simulink model "Vicon_Visualization"  (Simulink 9.1)
settings: Solver=FixedStepDiscrete  StartTime=0.0  StopTime=inf  FixedStep=0.001  RelTol=1e-3  EnableMultiTasking=on
undefined symbols (not defined in the file): localhost
libraries: quarc_library x6
settings Model: Creator=glai  LastModifiedBy=user  SimulationMode=external  ExtModeTrigDuration=5000
settings SolverCC: PositivePriorityOrder=on
settings DataIOCC: LimitDataPoints=on
settings OptimizationCC: LifeSpan=auto
settings DebuggingCC: UnderspecifiedInitializationDetection=Simplified  MergeDetectMultiDrivingBlocksExec=error  SolverPrmCheckMsg=warning
settings HardwareCC: ProdBitPerPointer=64  ProdBitPerSizeT=64  ProdBitPerPtrDiffT=64  ProdLargestAtomicFloat=Float  ProdIntDivRoundTo=Zero  ProdEndianess=LittleEndian  ProdWordSize=64  ProdHWDeviceType=Intel->x86-64 (Windows64)
settings RTWCC: Description=QUARC Win64 Target Using Toolchain  SystemTargetFile=quarc_win64.tlc  TemplateMakefile=quarc_default_tmf  Toolchain=QUARC win64 | nmake (64-bit Windows)  BuildConfiguration=Faster Runs
settings STFCustomTargetCC: ConcurrentExecutionCompliant=on  UseToolchainInfoCompliant=on  SystemTargetFile=quarc_win64.tlc
settings GRTTargetCC: ParMdlRefBuildCompliant=off  CompOptLevelCompliant=off  MatFileLogging=off  CPPClassGenCompliant=off  ExtMode=on  ExtModeMexFile=quarc_comm  ExtModeMexArgs='-w -d %d -uri %u', 'shmem://%m:1?timeout=10'
settings ConfigComp: CovSFcnEnable=off

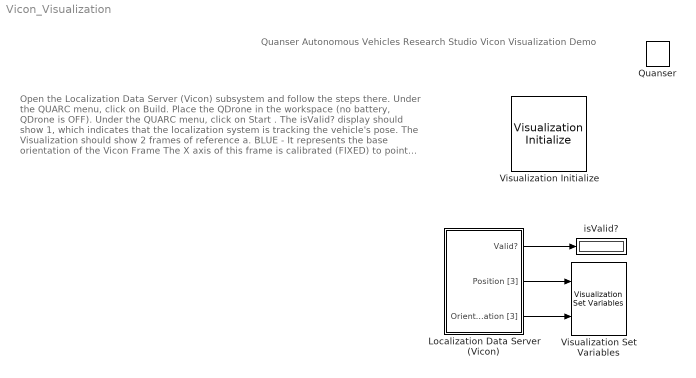
== system Vicon_Visualization ==
  note: Quanser Autonomous Vehicles Research Studio
      | Vicon Visualization Demo
  note: Open the Localization Data Server (Vicon) subsystem and follow the steps there.
      |
      | Under the QUARC menu, click on Build.
      |
      | Place the QDrone in the workspace (no battery, QDrone is OFF).
      |
      | Under the QUARC menu, click on Start .
      |
      | The isValid? display should show 1, which indicates that the localization system is tracking the vehicle's pose.
      |
      | The Visualization should show 2 frames of reference
      | a. BLUE - It represents the base orientation of the Vicon Frame
      | The X axis of this frame is calibrated (FIXED) to point away from the
      | ground control station PC. It is the same as the Research Studio Frame (RSF).
      |
      | b. RED - It represents the position and orientation of the QDrone's Body-Fixed Reference Frame as measured by Vicon data directly.
      |
      | When the vehicle is located at the workspace origin with 0 orientation (i.e., 0 Roll, 0 Pitch and 0 Yaw), the vehicle Body-Fixed Reference Frame will align with the Research Studio Frame (BLUE Basis Arrows).
      |
      | Step into the workspace and move the QDrone around by hand. The RED frame should move as it is Body-Fixed w.r.t. the QDrone.
      | NOTE : Hold the QDrone using the handle provided on the top frame
      |
      | Stop the model when finished.
  "Localization Data Server (Vicon) " : Subsystem
  Quanser : quarc_library/Logos/Quanser
  Visualization Initialize : quarc_library/User Interface/Visualization/Visualization Initialize  object_name=POSE_Check  scene_file=POSE_Check.xml  uri={'normal','';'Configuration','shmem://%m:2';}  apply_uri_to_all_configs=off  server_send_size=1000000  server_receive_size=1000  derive_from_server=on  client_send_size=1000  client_receive_size=1000000  variables=[ 60 61 80 81 ]  initial_values=single([ 0 0 0 0 0 0 0 0 0 0 0 0 ])  open_on_start=on  close_on_stop=on
      settings: AttributesFormatString=%<object_name>  SourceProductName=QUARC Targets
  Visualization Set Variables : quarc_library/User Interface/Visualization/Visualization Set Variables  object_name=POSE_Check  offset=[ 0 0 ]  data_type=[ 0 0 ]  length=[ 1 1 ]  sample_time=visualization_get_frame_period  actor_name={'actor.RefFrame.BodyFixed.OptiTrack/Position';'actor.RefFrame.BodyFixed.OptiTrack/Orientation'}
      settings: AttributesFormatString=(%<object_name>)  SourceProductName=QUARC Targets
  isValid? : Display
  wires:
  "Localization Data Server (Vicon) "/2(Position [3]) -> Visualization Set Variables/1
  "Localization Data Server (Vicon) "/3(Orientation [3]) -> Visualization Set Variables/2
  "Localization Data Server (Vicon) "/1(Valid?) -> isValid?/1

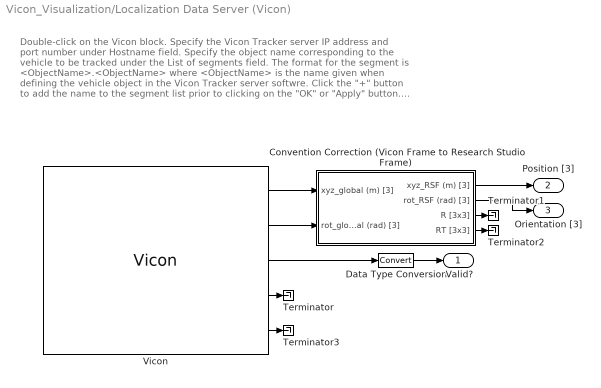
== system Vicon_Visualization/Localization Data Server (Vicon)  ==
  note: Double-click on the Vicon block.
      |
      | Specify the Vicon Tracker server IP address and port number under Hostname field.
      |
      | Specify the object name corresponding to the vehicle to be tracked under the
      | List of segments field. The format for the segment is <ObjectName>.<ObjectName>
      | where <ObjectName> is the name given when defining the vehicle object in the
      | Vicon Tracker server softwre. Click the "+" button to add the name to the segment list
      | prior to clicking on the "OK" or "Apply" button.
      | Remove extra/unused entries from the list using the "-" button.
  Convention Correction (Vicon Frame to Research Studio Frame) : Subsystem
  Data Type Conversion : DataTypeConversion
  Terminator{,1..3} (4 alike) : Terminator
  Vicon : quarc_library/Devices/Third-Party/Vicon/Vicon  hostname=localhost:801  segment_list=ObjectName1.ObjectName1\0\0  marker_list=\0  unlabeled_markers=[]  stream_mode=2  sample_time=qc_get_step_size  num_segments=1  num_markers=0  active=on
      settings: SourceProductName=QUARC Targets
  Valid? : Outport  VectorParamsAs1DForOutWhenUnconnected=off
  Position [3] : Outport  Port=2  VectorParamsAs1DForOutWhenUnconnected=off
  Orientation [3] : Outport  Port=3  VectorParamsAs1DForOutWhenUnconnected=off
  wires:
  Vicon/3 -> Data Type Conversion/1
  Data Type Conversion/1 -> Valid?/1
  Convention Correction (Vicon Frame to Research Studio Frame)/1(xyz_RSF (m) [3]) -> Position [3]/1
  Convention Correction (Vicon Frame to Research Studio Frame)/2(rot_RSF (rad) [3]) -> Orientation [3]/1
  Convention Correction (Vicon Frame to Research Studio Frame)/3(R [3x3]) -> Terminator1/1
  Convention Correction (Vicon Frame to Research Studio Frame)/4(RT [3x3]) -> Terminator2/1
  Vicon/1 -> Convention Correction (Vicon Frame to Research Studio Frame)/1(xyz_global (m) [3])
  Vicon/2 -> Convention Correction (Vicon Frame to Research Studio Frame)/2(rot_global (rad) [3])
  Vicon/4 -> Terminator/1
  Vicon/5 -> Terminator3/1

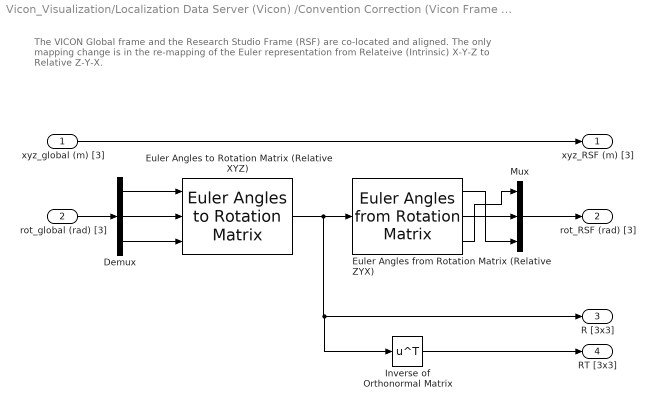
== system Vicon_Visualization/Localization Data Server (Vicon) /Convention Correction (Vicon Frame to Research Studio Frame) ==
  note: The VICON Global frame and the Research Studio Frame (RSF) are co-located and aligned.
      | The only mapping change is in the re-mapping of the Euler representation from
      | Relateive (Intrinsic) X-Y-Z to Relative Z-Y-X.
  xyz_global (m) [3] : Inport
  rot_global (rad) [3] : Inport  Port=2
  Demux : Demux  Outputs=3
  Euler Angles from Rotation Matrix (Relative ZYX) : quarc_library/Math Operations/Matrices/Euler Angles from Rotation Matrix  menu_order=Relative Z-Y-X
      settings: SourceProductName=QUARC Targets
  Euler Angles to Rotation Matrix (Relative XYZ) : quarc_library/Math Operations/Matrices/Euler Angles to Rotation Matrix  menu_order=Relative X-Y-Z
      settings: SourceProductName=QUARC Targets
  Inverse of Orthonormal Matrix : Math  Operator=transpose  SaturateOnIntegerOverflow=on
  Mux : Mux  Inputs=3
  xyz_RSF (m) [3] : Outport  VectorParamsAs1DForOutWhenUnconnected=off
  rot_RSF (rad) [3] : Outport  Port=2  VectorParamsAs1DForOutWhenUnconnected=off
  R [3x3] : Outport  Port=3  VectorParamsAs1DForOutWhenUnconnected=off
  RT [3x3] : Outport  Port=4  VectorParamsAs1DForOutWhenUnconnected=off
  wires:
  Demux/3 -> Euler Angles to Rotation Matrix (Relative XYZ)/3
  Demux/1 -> Euler Angles to Rotation Matrix (Relative XYZ)/1
  rot_global (rad) [3]/1 -> Demux/1
  Demux/2 -> Euler Angles to Rotation Matrix (Relative XYZ)/2
  xyz_global (m) [3]/1 -> xyz_RSF (m) [3]/1
  Euler Angles from Rotation Matrix (Relative ZYX)/1 -> Mux/3
  Mux/1 -> rot_RSF (rad) [3]/1
  Euler Angles from Rotation Matrix (Relative ZYX)/3 -> Mux/1
  Euler Angles from Rotation Matrix (Relative ZYX)/2 -> Mux/2
  Euler Angles to Rotation Matrix (Relative XYZ)/1 -> Inverse of Orthonormal Matrix/1, R [3x3]/1, Euler Angles from Rotation Matrix (Relative ZYX)/1
  Inverse of Orthonormal Matrix/1 -> RT [3x3]/1
